simulink model "RecoveryCurrent_ExternalFault"  (R2015a)
settings: Solver=ode45  StartTime=0.0  StopTime=1  RelTol=1e-3
undefined symbols (not defined in the file or in its folder): D11, Delta
libraries: powerlib x16
settings Model: Creator=baishuhua  LastModifiedBy=baishuhua
settings DebuggingCC: AlgebraicLoopMsg=none

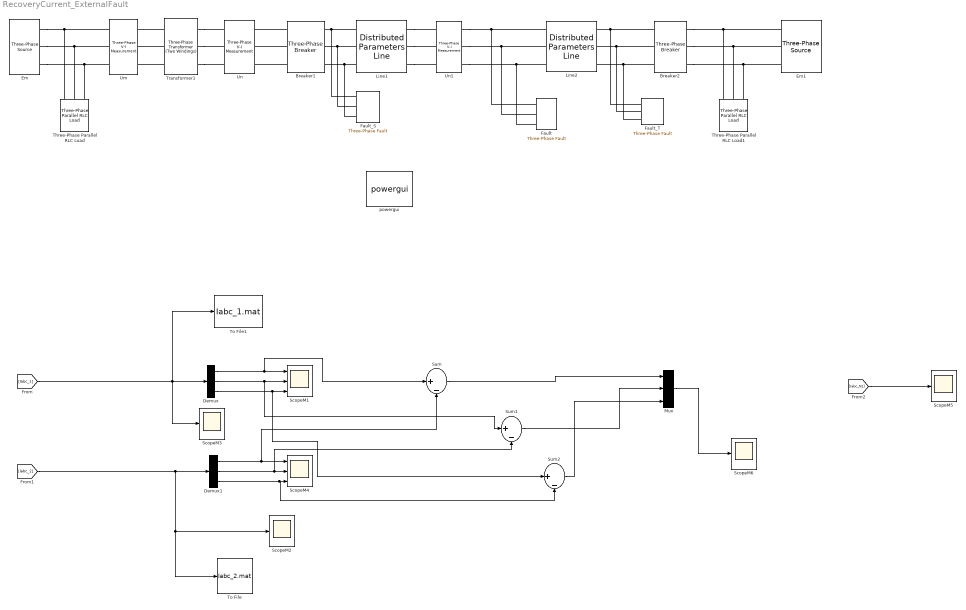
== system RecoveryCurrent_ExternalFault ==
  Breaker1 : powerlib/Elements/Three-Phase Breaker  InitialState=closed  SwitchA=on  SwitchB=on  SwitchC=on  SwitchTimes=[0.36 0.86]  External=off  BreakerResistance=0.01  SnubberResistance=1e6  SnubberCapacitance=inf  Measurements=None
  Breaker2 : powerlib/Elements/Three-Phase Breaker  InitialState=closed  SwitchA=on  SwitchB=on  SwitchC=on  SwitchTimes=[0.36 0.86]  External=off  BreakerResistance=0.01  SnubberResistance=1e6  SnubberCapacitance=inf  Measurements=None
  Demux : Demux  Outputs=3
  Demux1 : Demux  Outputs=3
  Em : powerlib/Electrical Sources/Three-Phase Source  Voltage=220e3  PhaseAngle=30  Frequency=50  InternalConnection=Yg  SpecifyImpedance=off  Resistance=0.8929  Inductance=0.05  ShortCircuitLevel=100e6  BaseVoltage=220e3  XRratio=7  BusType=swing  Pref=0  Qref=0  Qmin=-inf  Qmax=inf
  Em1 : powerlib/Electrical Sources/Three-Phase Source  Voltage=500e3  PhaseAngle=10  Frequency=50  InternalConnection=Yg  SpecifyImpedance=off  Resistance=0.8929  Inductance=0.05  ShortCircuitLevel=100e6  BaseVoltage=500e3  XRratio=7  BusType=swing  Pref=0  Qref=0  Qmin=-inf  Qmax=inf
  Fault : powerlib/Elements/Three-Phase Fault  InitialStates=0  FaultA=on  FaultB=off  FaultC=on  GroundFault=off  SwitchTimes=[10.3 10.36]  External=off  SwitchStatus=NaN  FaultResistance=0.001  GroundResistance=0.01  SnubberResistance=1e6  SnubberCapacitance=inf  Measurements=None
  Fault_S : powerlib/Elements/Three-Phase Fault  InitialStates=0  FaultA=on  FaultB=off  FaultC=on  GroundFault=off  SwitchTimes=[10.3 10.36]  External=off  SwitchStatus=NaN  FaultResistance=0.001  GroundResistance=0.01  SnubberResistance=1e6  SnubberCapacitance=inf  Measurements=None
  Fault_T : powerlib/Elements/Three-Phase Fault  InitialStates=0  FaultA=on  FaultB=off  FaultC=on  GroundFault=off  SwitchTimes=[0.3 0.36]  External=off  SwitchStatus=NaN  FaultResistance=0.001  GroundResistance=0.01  SnubberResistance=1e6  SnubberCapacitance=inf  Measurements=None
  Line1 : powerlib/Elements/Distributed Parameters Line  Phases=3  Frequency=50  Resistance=[0.01273 0.3864]  Inductance="[0.9337e-3  4.1264e-3]"  Capacitance=[12.74e-9 7.751e-9]  Length=120  x1=[-0.0007 -1.21220953958105e-07 0 0;-0.0006 -1.19925674909227e-07 0 0;-0.0005 -1.18512043698015e-07 300198.054562506 -413899.704998335;-0.0004 -1.16981455407806e-07 313050.828860466 -404266.021711691;-0.0003 -1.15335420544451e-07 325594.659785425 -394233.376669246;-0.0002 -1.13575563545634e-07 337817.168090695 -383811.670880402;-0.0001 -1.1170362117774e-07 349706.291636221 -373011.189310542]  x2=[-0.0007 -9.15624609766372e-08 0 0;-0.0006 -9.0061871113903e-08 0 0;-0.0005 -8.84724010576808e-08 283485.743646309 -426249.02442062;-0.0004 -8.67956194230171e-08 296734.665958007 -417134.193862144;-0.0003 -8.50331809909449e-08 309690.746979615 -407607.702215548;-0.0002 -8.31868250754151e-08 322341.200623371 -397678.95097794;-0.0001 -8.1258373806803e-08 334673.542418837 -387357.738628078]  x3=[-0.0007 -1.53864474143839e-10 0 0;-0.0006 -1.46946530301084e-10 0 0;-0.0005 -1.39883567973991e-10 634.275353953178 -1135.66169238899;-0.0004 -1.32682557453655e-10 669.634373168382 -1115.17824156663;-0.0003 -1.25350605268072e-10 704.332544103206 -1093.59424445695;-0.0002 -1.17894947168852e-10 738.3356238521 -1070.93100185922;-0.0001 -1.10322940990405e-10 771.610055480591 -1047.21087965772]  x4=[-0.0007 -1.37910574604727e-10 0 0;-0.0006 -1.42043546781659e-10 0 0;-0.0005 -1.46036339127043e-10 1311.18628581732 -2094.58307462023;-0.0004 -1.49885011236889e-10 1376.33173886202 -2052.36416778359;-0.0003 -1.53585764936482e-10 1440.118918647 -2008.11982529827;-0.0002 -1.57134948028716e-10 1502.48487492695 -1961.89371098863;-0.0001 -1.60529057898378e-10 1563.36806003254 -1913.73144444854]  x5=0.000678649880394891  V1=[1.631e-09 2.327e+05 2.327e+05;314.2 314.2 314.2;-0.2328 1.279 -0.2922]  V2=[1.314e-09 2.279e+05 2.279e+05;314.2 314.2 314.2;-0.1643 1.215 -0.3554]  I1=[9.953e-12 946.9 946.9;314.2 314.2 314.2;0.9625 -2.43 2.283]  I2=[7.788e-12 2564 2564;314.2 314.2 314.2;-1.449 1.047 -0.524]  nHarmo=1  Measurements=None
  Line2 : powerlib/Elements/Distributed Parameters Line  Phases=3  Frequency=50  Resistance=[0.01273 0.3864]  Inductance="[0.9337e-3  4.1264e-3]"  Capacitance=[12.74e-9 7.751e-9]  Length=120  x1=[-0.0007 -9.15624609766372e-08 0 0;-0.0006 -9.0061871113903e-08 0 0;-0.0005 -8.84724010576808e-08 283485.743646309 -426249.02442062;-0.0004 -8.67956194230171e-08 296734.665958007 -417134.193862144;-0.0003 -8.50331809909449e-08 309690.746979615 -407607.702215548;-0.0002 -8.31868250754151e-08 322341.200623371 -397678.95097794;-0.0001 -8.1258373806803e-08 334673.542418837 -387357.738628078]  x2=[-0.0007 -8.4140908256497e-09 0 0;-0.0006 -8.21656592460417e-09 0 0;-0.0005 -8.01093226498909e-09 262314.826129681 -431185.633023829;-0.0004 -7.79739278240003e-09 275729.257634674 -422733.361136588;-0.0003 -7.57615821452539e-09 288871.577651578 -413863.902459121;-0.0002 -7.34744689317368e-09 301728.816297228 -404586.010076322;-0.0001 -7.11148452880642e-09 314288.285029355 -394908.840147839]  x3=[-0.0007 2.48047323585325e-10 0 0;-0.0006 2.62386528806871e-10 0 0;-0.0005 2.76466790202795e-10 774.570131637061 -1041.55924662667;-0.0004 2.90274212255028e-10 806.904094595971 -1016.71546421898;-0.0003 3.03795168704995e-10 838.441740632226 -990.868306397658;-0.0002 3.17016316001086e-10 869.151945896776 -964.0432811869;-0.0001 3.29924606467128e-10 899.004403124712 -936.266861647967]  x4=[-0.0007 -3.86442291992462e-10 0 0;-0.0006 -3.99010448476311e-10 0 0;-0.0005 -4.11184829820628e-10 1027.40238525913 -2243.18285925816;-0.0004 -4.22953421380859e-10 1097.35550056225 -2209.80449512881;-0.0003 -4.34304608977972e-10 1166.22565847165 -2174.24532075571;-0.0002 -4.45227190360255e-10 1233.94489245627 -2136.54042875083;-0.0001 -4.55710386258582e-10 1300.44637180801 -2096.72702929044]  x5=0.000678649880394891  V1=[1.314e-09 2.279e+05 2.279e+05;314.2 314.2 314.2;-0.4841 1.02 -0.5504]  V2=[3.97e-10 2.167e+05 2.167e+05;314.2 314.2 314.2;0.3474 0.5318 -1.039]  I1=[3.773e-12 946.7 946.7;314.2 314.2 314.2;0.6255 -2.591 2.121]  I2=[3.658e-12 2534 2534;314.2 314.2 314.2;-1.915 0.6244 -0.9464]  nHarmo=1  Measurements=None
  Mux : Mux  Inputs=3
  ScopeM1 : Scope  NumInputPorts=3
      settings: ShowLegends=on  TimeRange=2  YMin=-1250~-1250~-1250  YMax=1250~1250~1250  SampleInput=on
  ScopeM{2..3,5..6} (4 alike) : Scope
      ScopeM2 settings: ShowLegends=on  TimeRange=10  YMin=-500  YMax=4000  SaveName=ScopeData2  SampleInput=on
      ScopeM3 settings: ShowLegends=on  TimeRange=10  YMin=-10  YMax=15  SaveName=ScopeData3  SampleInput=on
      ScopeM5 settings: ShowLegends=on  TimeRange=10  YMin=-500  YMax=4000  SaveName=ScopeData4  SampleInput=on
      ScopeM6 settings: ShowLegends=on  TimeRange=10  YMin=-500  YMax=4000  SaveName=ScopeData5  SampleInput=on
  ScopeM4 : Scope  NumInputPorts=3
      settings: ShowLegends=on  TimeRange=10  YMin=-500~-5~-5  YMax=4000~5~5  SampleInput=on
  Sum : Sum  Inputs=|+-
  Sum1 : Sum  Inputs=|+-
  Sum2 : Sum  Inputs=|+-
  Three-Phase Parallel RLC Load : powerlib/Elements/Three-Phase Parallel RLC Load  LConnTagsString=A|B|C  Configuration=Y (grounded)  NominalVoltage=220e3  NominalFrequency=50  ActivePower=10e6  InductivePower=100  CapacitivePower=100  Measurements=None  LoadType=constant PQ
  Three-Phase Parallel RLC Load1 : powerlib/Elements/Three-Phase Parallel RLC Load  LConnTagsString=A|B|C  Configuration=Y (grounded)  NominalVoltage=500e3  NominalFrequency=50  ActivePower=200e6  InductivePower=100  CapacitivePower=100  Measurements=None  LoadType=constant PQ
  To File : ToFile  Filename=Iabc_2.mat  MatrixName=Iabc_2  SaveFormat=Timeseries
  To File1 : ToFile  Filename=Iabc_1.mat  MatrixName=Iabc_1  SaveFormat=Timeseries
  Transformer1 : powerlib/Elements/Three-Phase Transformer (Two Windings)  Winding1Connection=Delta (D11)  Winding2Connection=Delta (D11)  CoreType=Three single-phase transformers  SetSaturation=on  Hysteresis=off  DataFile='hysteresis'  SetInitialFlux=on  Measurements=None  UNITS=pu  NominalPower=[ 300e6 , 50 ]  Winding1=[ 220e3 , 0.002 , 0.08 ]  Winding2=[ 500e3 , 0.002 , 0.08 ]  Rm=500  Lm=500  L0=0.5  Saturation=[ 0,0 ; 0.0024,1.2 ; 1.0,1.52 ]  InitialFluxes=[0.2 -0.3 0.3]  MoreParameters=off  BreakLoop=off  DataType=off  TransfoNumber=1
  Um : powerlib/Measurements/Three-Phase V-I Measurement  VoltageMeasurement=no  SetLabelV=on  LabelV=Vabc_M  Vpu=off  VpuLL=off  CurrentMeasurement=yes  SetLabelI=on  LabelI=Iabc_1  Ipu=on  Pbase=300e6  Vbase=220e3  OutputType=Complex  PhasorSimulation=off  PSBequivalent=0
  Un : powerlib/Measurements/Three-Phase V-I Measurement  VoltageMeasurement=no  SetLabelV=on  LabelV=Vabc_M  Vpu=off  VpuLL=off  CurrentMeasurement=yes  SetLabelI=on  LabelI=Iabc_2  Ipu=on  Pbase=300e6  Vbase=500e3  OutputType=Complex  PhasorSimulation=off  PSBequivalent=0
  Un1 : powerlib/Measurements/Three-Phase V-I Measurement  VoltageMeasurement=no  SetLabelV=on  LabelV=Vabc_M  Vpu=off  VpuLL=off  CurrentMeasurement=yes  SetLabelI=on  LabelI=Iabc_N1  Ipu=on  Pbase=100e6  Vbase=500e3  OutputType=Complex  PhasorSimulation=off  PSBequivalent=0
  powergui : powerlib/powergui  Priority=1  SimulationMode=Discrete  SolverType=Tustin  SampleTime=1e-4  frequency=60  SPID=off  DisableSnubberDevices=off  DisableRonSwitches=off  DisableVfSwitches=off  SwTol=0  DisplayEquations=off  Interpol=off  methode=off  Ts=0  FunctionMessages=off  echomessages=off  HookPort=off  EnableUseOfTLC=off  x0status=blocks  frequencyindice=50  Pbase=100e6  ErrMax=1e-4  Iterations=50  UnitsV=kV  UnitsW=MW  buscounter=0  RestoreLinks=warning  ResistiveCurrentMeasurement=off  Frange=[0:2:500]  Ylog=off  Xlog=on  ShowGrid=off  save=off  variable=ZData  structure=ScopeData  ZoomFFT=off  StartTime=0.191  cycles=2  DisplayStyle=5  fundamental=50  FreqAxis=on  MaxFrequency=250  frequencyindicesteady=1  RmsSteady=1  display=off
  wires:
  [Iabc_1] -> To File1/1, ScopeM3/1, Demux/1
  Demux/1 -> ScopeM1/1, Sum/1
  Demux/2 -> ScopeM1/2, Sum1/1
  Demux/3 -> ScopeM1/3, Sum2/1
  Sum/1 -> Mux/1
  Sum1/1 -> Mux/2
  Sum2/1 -> Mux/3
  Mux/1 -> ScopeM6/1
  Demux1/1 -> Sum/2, ScopeM4/1
  Demux1/2 -> Sum1/2, ScopeM4/2
  Demux1/3 -> Sum2/2, ScopeM4/3
  [Iabc_N1] -> ScopeM5/1
  [Iabc_2] -> Demux1/1, To File/1, ScopeM2/1
  connections:
  Three-Phase Parallel RLC Load/LConn1 -- Em/RConn1 -- Um/LConn1
  Em/RConn2 -- Three-Phase Parallel RLC Load/LConn2 -- Um/LConn2
  Em/RConn3 -- Three-Phase Parallel RLC Load/LConn3 -- Um/LConn3
  Transformer1/LConn1 -- Um/RConn1
  Transformer1/LConn2 -- Um/RConn2
  Transformer1/LConn3 -- Um/RConn3
  Em1/RConn1 -- Breaker2/RConn1 -- Three-Phase Parallel RLC Load1/LConn1
  Breaker2/LConn1 -- Fault_T/LConn1 -- Line2/RConn1
  Breaker2/LConn2 -- Fault_T/LConn2 -- Line2/RConn2
  Breaker2/LConn3 -- Fault_T/LConn3 -- Line2/RConn3
  Transformer1/RConn1 -- Un/LConn1
  Transformer1/RConn2 -- Un/LConn2
  Transformer1/RConn3 -- Un/LConn3
  Breaker1/LConn1 -- Un/RConn1
  Breaker1/LConn2 -- Un/RConn2
  Breaker1/LConn3 -- Un/RConn3
  Un1/RConn1 -- Fault/LConn1 -- Line2/LConn1
  Un1/RConn2 -- Fault/LConn2 -- Line2/LConn2
  Un1/RConn3 -- Fault/LConn3 -- Line2/LConn3
  Line1/LConn1 -- Fault_S/LConn1 -- Breaker1/RConn1
  Line1/LConn2 -- Fault_S/LConn2 -- Breaker1/RConn2
  Line1/LConn3 -- Fault_S/LConn3 -- Breaker1/RConn3
  Em1/RConn2 -- Breaker2/RConn2 -- Three-Phase Parallel RLC Load1/LConn2
  Em1/RConn3 -- Breaker2/RConn3 -- Three-Phase Parallel RLC Load1/LConn3
  Line1/RConn1 -- Un1/LConn1
  Line1/RConn2 -- Un1/LConn2
  Line1/RConn3 -- Un1/LConn3
